simulink model "DelaySimulation"  (R2019a)
settings: Solver=ode45  StartTime=0.0  StopTime=70  RelTol=1e-3  EnableMultiTasking=on
settings Model: Creator=Owner  LastModifiedBy=PC
settings DataIOCC: LimitDataPoints=on  SaveFormat=Array  ReturnWorkspaceOutputs=off
settings OptimizationCC: LifeSpan=inf
settings DebuggingCC: SolverPrmCheckMsg=warning  SFUnexpectedBacktrackingDiag=warning  SFNoUnconditionalDefaultTransitionDiag=warning  SFExecutionAtInitializationDiag=none  ArithmeticOperatorsInVariantConditions=warning
settings HardwareCC: ProdBitPerPointer=32  ProdBitPerSizeT=32  ProdBitPerPtrDiffT=32  ProdLargestAtomicFloat=None  ProdIntDivRoundTo=Undefined  ProdEndianess=Unspecified  ProdWordSize=32  ProdHWDeviceType=32-bit Generic
settings ModelReferenceCC: PropagateSignalLabelsOutOfModel=off
settings SFSimCC: SimUseLocalCustomCode=off
settings RTWCC: RTWUseLocalCustomCode=off
settings CodeAppCC: StateflowObjectComments=on
settings GRTTargetCC: TargetLangStandard=C89/C90 (ANSI)  GeneratePreprocessorConditionals=Disable all
settings ConfigComp: CovMetricSettings=dw  CovHtmlReporting=on  CovSaveCumulativeToWorkspaceVar=on  CovSaveSingleToWorkspaceVar=on  CovExternalEMLEnable=off  CovSFcnEnable=off

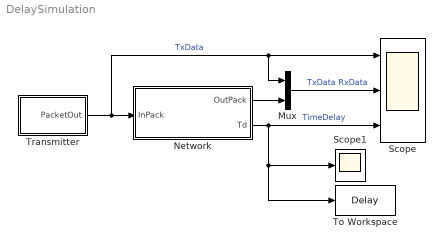
== system DelaySimulation ==
  Mux : Mux  Inputs=2
  Network : Subsystem
  Scope : Scope  NumInputPorts=3
  Scope1 : Scope
  To Workspace : ToWorkspace  VariableName=Delay  SampleTime=-1
  Transmitter : Subsystem
  wires:
  Network/2(Td) -> Scope/3, To Workspace/1, Scope1/1  "TimeDelay"
  Network/1(OutPack) -> Mux/2
  Mux/1 -> Scope/2  "TxData RxData"
  Transmitter/1(PacketOut) -> Scope/1, Mux/1, Network/1(InPack)  "TxData"

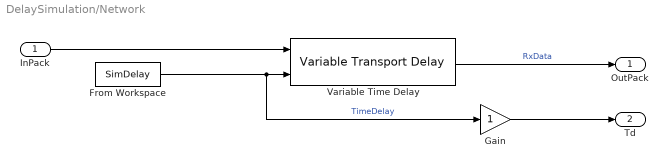
== system DelaySimulation/Network ==
  InPack : Inport
  From Workspace : FromWorkspace  VariableName=SimDelay  OutDataTypeStr=double  SampleTime=0
  Gain : Gain
  Variable Time Delay : VariableTransportDelay  MaximumDelay=10
  OutPack : Outport
  Td : Outport  Port=2
  wires:
  From Workspace/1 -> Gain/1, Variable Time Delay/2  "TimeDelay"
  Variable Time Delay/1 -> OutPack/1  "RxData"
  InPack/1 -> Variable Time Delay/1
  Gain/1 -> Td/1

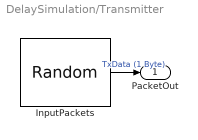
== system DelaySimulation/Transmitter ==
  InputPackets : UniformRandomNumber  Minimum=-128  Maximum=127  SampleTime=0.1
  PacketOut : Outport
  wires:
  InputPackets/1 -> PacketOut/1  "TxData (1 Byte)"
